simulink model "zbiorniki"  (Simulink 8.4)
settings: Solver=ode45  StartTime=0.0  StopTime=10.0  RelTol=1e-3
values from neighbouring files (symbols this model uses):
  a = 10    [lab.m]    (also in rhs2.m; rhs3.m; zbiornik2.m; zbiorniki.m)
  a1 = 0.5    [lab.m]    (also in rhs2.m; rhs3.m; zbiornik2.m; zbiorniki.m)
  a2 = 0.5    [lab.m]    (also in rhs2.m; rhs3.m; zbiornik2.m; zbiorniki.m)
  a3 = 0.5    [lab.m]    (also in rhs2.m; rhs3.m; zbiornik2.m; zbiorniki.m)
  b = 44.5    [lab.m]    (also in rhs2.m; rhs3.m; zbiornik2.m; zbiorniki.m)
  c = 25    [lab.m]    (also in rhs2.m; rhs3.m; zbiornik2.m; zbiorniki.m)
  c1 = 19.01    [lab.m]    (also in rhs2.m; rhs3.m; zbiornik2.m; zbiorniki.m)
  c2 = 32.45    [lab.m]    (also in rhs2.m; rhs3.m; zbiornik2.m; zbiorniki.m)
  c3 = 32.45    [lab.m]    (also in rhs2.m; rhs3.m; zbiornik2.m; zbiorniki.m)
  H = 35    [lab.m]    (also in rhs2.m; rhs3.m; zbiornik2.m; zbiorniki.m)
  R = 36.4    [lab.m]    (also in rhs2.m; rhs3.m; zbiornik2.m; zbiorniki.m)
  w = 3.5    [lab.m]    (also in rhs2.m; rhs3.m; zbiornik2.m; zbiorniki.m)
settings Model: Creator=Jadwiga Piechota  LastModifiedBy=Jadwiga Piechota
settings DataIOCC: SignalLoggingSaveFormat=Dataset
settings OptimizationCC: ExpressionDepthLimit=128
settings DebuggingCC: UnderspecifiedInitializationDetection=Simplified  MergeDetectMultiDrivingBlocksExec=error  FcnCallInpInsideContextMsg=EnableAllAsError  StateNameClashWarn=none
settings GRTTargetCC: CombineOutputUpdateFcns=on  GRTInterface=off

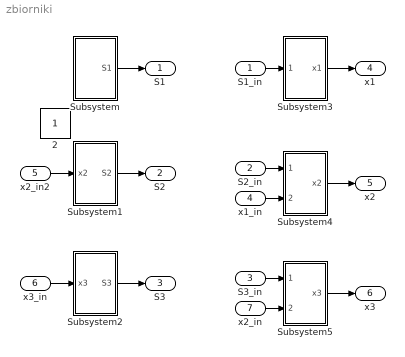
== system zbiorniki ==
  S1_in : Inport
  S2_in : Inport  Port=2
  S3_in : Inport  Port=3
  x1_in : Inport  Port=4
  x2_in2 : Inport  Port=5
  x3_in : Inport  Port=6
  x2_in : Inport  Port=7
  Subsystem : Subsystem
  Subsystem1 : Subsystem
  Subsystem2 : Subsystem
  Subsystem3 : Subsystem
  Subsystem4 : Subsystem
  Subsystem5 : Subsystem
  S1 : Outport
  S2 : Outport  Port=2
  S3 : Outport  Port=3
  x1 : Outport  Port=4
  x2 : Outport  Port=5
  x3 : Outport  Port=6
  2 : Constant  IOType=siggen
  wires:
  Subsystem/1(S1) -> S1/1
  S1_in/1 -> Subsystem3/1(S1_in)
  Subsystem3/1(x1) -> x1/1
  S2_in/1 -> Subsystem4/1(S2_in)
  x1_in/1 -> Subsystem4/2(x1_in)
  Subsystem4/1(x2) -> x2/1
  S3_in/1 -> Subsystem5/1(S3_in)
  x2_in/1 -> Subsystem5/2(x2_in)
  Subsystem5/1(x3) -> x3/1
  Subsystem1/1(S2) -> S2/1
  x2_in2/1 -> Subsystem1/1(x2)
  Subsystem2/1(S3) -> S3/1
  x3_in/1 -> Subsystem2/1(x3)

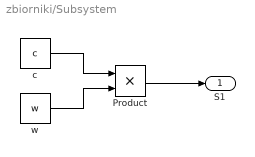
== system zbiorniki/Subsystem ==
  Product : Product
  c : Constant  Value=c
  w : Constant  Value=w
  S1 : Outport
  wires:
  Product/1 -> S1/1
  c/1 -> Product/1
  w/1 -> Product/2

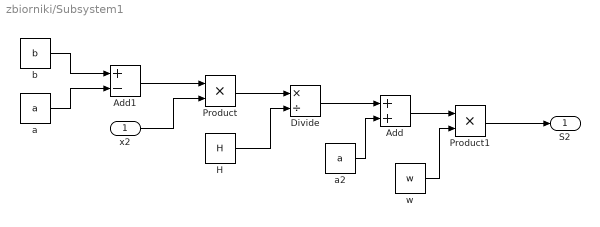
== system zbiorniki/Subsystem1 ==
  x2 : Inport
  Add : Sum
  Add1 : Sum  Inputs=+-
  Divide : Product  Inputs=*/
  H : Constant  Value=H
  Product : Product
  Product1 : Product
  a : Constant  Value=a
  a2 : Constant  Value=a
  b : Constant  Value=b
  w : Constant  Value=w
  S2 : Outport
  wires:
  Product/1 -> Divide/1
  Divide/1 -> Add/1
  Add/1 -> Product1/1
  Product1/1 -> S2/1
  x2/1 -> Product/2
  b/1 -> Add1/1
  Add1/1 -> Product/1
  a/1 -> Add1/2
  w/1 -> Product1/2
  a2/1 -> Add/2
  H/1 -> Divide/2

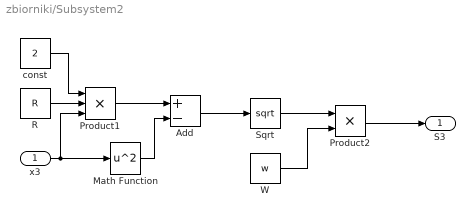
== system zbiorniki/Subsystem2 ==
  x3 : Inport
  Add : Sum  Inputs=+-
  Math Function : Math  Operator=square  SaturateOnIntegerOverflow=on
  Product1 : Product  Inputs=3
  Product2 : Product
  R : Constant  Value=R
  Sqrt : Sqrt  SaturateOnIntegerOverflow=on
  W : Constant  Value=w
  const : Constant  Value=2
  S3 : Outport
  wires:
  Math Function/1 -> Add/2
  Product2/1 -> S3/1
  Product1/1 -> Add/1
  Sqrt/1 -> Product2/1
  W/1 -> Product2/2
  x3/1 -> Product1/3, Math Function/1
  Add/1 -> Sqrt/1
  const/1 -> Product1/1
  R/1 -> Product1/2

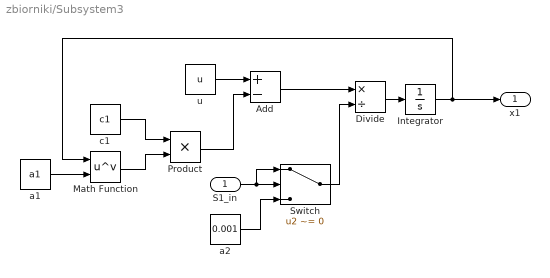
== system zbiorniki/Subsystem3 ==
  S1_in : Inport
  Add : Sum  Inputs=+-
  Divide : Product  Inputs=*/
  Integrator : Integrator
  Math Function : Math  Operator=pow  SaturateOnIntegerOverflow=on
  Product : Product
  Switch : Switch  Criteria=u2 ~= 0
  a1 : Constant  Value=a1
  a2 : Constant  Value=0.001
  c1 : Constant  Value=c1
  u : Constant  Value=u
  x1 : Outport
  wires:
  Math Function/1 -> Product/2
  Product/1 -> Add/2
  Divide/1 -> Integrator/1
  Integrator/1 -> x1/1, Math Function/1
  u/1 -> Add/1
  c1/1 -> Product/1
  Add/1 -> Divide/1
  a1/1 -> Math Function/2
  a2/1 -> Switch/3
  Switch/1 -> Divide/2
  S1_in/1 -> Switch/1, Switch/2

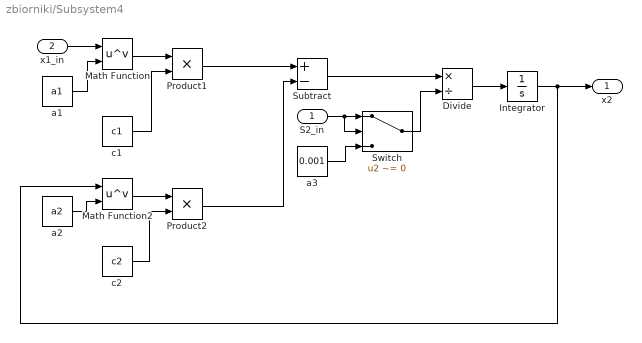
== system zbiorniki/Subsystem4 ==
  S2_in : Inport
  x1_in : Inport  Port=2
  Divide : Product  Inputs=*/
  Integrator : Integrator
  Math Function : Math  Operator=pow  SaturateOnIntegerOverflow=on
  Math Function2 : Math  Operator=pow  SaturateOnIntegerOverflow=on
  Product1 : Product
  Product2 : Product
  Subtract : Sum  Inputs=+-
  Switch : Switch  Criteria=u2 ~= 0
  a1 : Constant  Value=a1
  a2 : Constant  Value=a2
  a3 : Constant  Value=0.001
  c1 : Constant  Value=c1
  c2 : Constant  Value=c2
  x2 : Outport
  wires:
  x1_in/1 -> Math Function/1
  c1/1 -> Product1/2
  Integrator/1 -> x2/1, Math Function2/1
  a1/1 -> Math Function/2
  a2/1 -> Math Function2/2
  Math Function2/1 -> Product2/1
  c2/1 -> Product2/2
  Product2/1 -> Subtract/2
  Math Function/1 -> Product1/1
  Divide/1 -> Integrator/1
  Product1/1 -> Subtract/1
  Subtract/1 -> Divide/1
  a3/1 -> Switch/3
  S2_in/1 -> Switch/1, Switch/2
  Switch/1 -> Divide/2

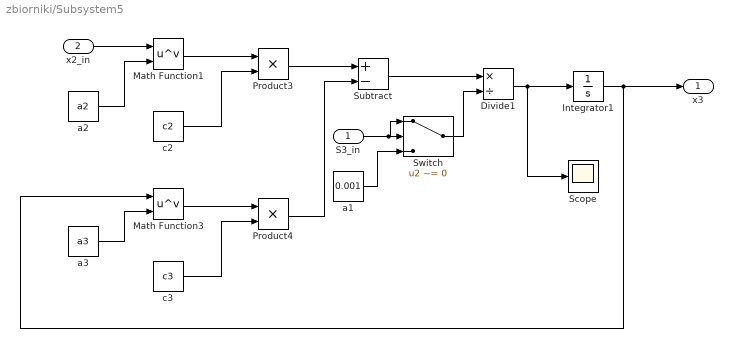
== system zbiorniki/Subsystem5 ==
  S3_in : Inport
  x2_in : Inport  Port=2
  Divide1 : Product  Inputs=*/
  Integrator1 : Integrator
  Math Function1 : Math  Operator=pow  SaturateOnIntegerOverflow=on
  Math Function3 : Math  Operator=pow  SaturateOnIntegerOverflow=on
  Product3 : Product
  Product4 : Product
  Scope : Scope
  Subtract : Sum  Inputs=+-
  Switch : Switch  Criteria=u2 ~= 0
  a1 : Constant  Value=0.001
  a2 : Constant  Value=a2
  a3 : Constant  Value=a3
  c2 : Constant  Value=c2
  c3 : Constant  Value=c3
  x3 : Outport
  wires:
  Product4/1 -> Subtract/2
  c2/1 -> Product3/2
  Product3/1 -> Subtract/1
  Math Function1/1 -> Product3/1
  Subtract/1 -> Divide1/1
  S3_in/1 -> Switch/1, Switch/2
  Math Function3/1 -> Product4/1
  a3/1 -> Math Function3/2
  Divide1/1 -> Scope/1, Integrator1/1
  c3/1 -> Product4/2
  Integrator1/1 -> x3/1, Math Function3/1
  x2_in/1 -> Math Function1/1
  a2/1 -> Math Function1/2
  a1/1 -> Switch/3
  Switch/1 -> Divide1/2
